simulink model "active_suspension_sim"  (R2020a)
settings: Solver=ode45  StartTime=0.0  StopTime=10.0  RelTol=1e-3
values from neighbouring files (symbols this model uses):
  A = [[-1/tau 0];[1/m -rho*CD*Af*x2e/m]]    [CruiseCtrl_StateFeedback_Int_design.m]    (also in CruiseCtrl_StateFeedback_Int_design_EJ6.m = Aaug; Driveline_ctrl_design.m = [-ds/(Jf*i^2) ds/(Jf*i) -cs/(Jf*i); Driveline_ctrl_design_accion_int.m = [-ds/(Jf*i^2) ds/(Jf*i) -cs/(Jf*i); active_suspension_ctrl_design.m = [[0 1 0 0 0];[-(cw+cs)/mw -ds/mw cs/mw ds/mw -1/mw];[0 0 0 1)
  B1 = [B H]    [CruiseCtrl_StateFeedback_Int_design.m]    (also in CruiseCtrl_StateFeedback_Int_design_EJ6.m = [Baug Haug]; Driveline_ctrl_design.m; Driveline_ctrl_design_accion_int.m; active_suspension_ctrl_design.m)
  C = [0 1]    [CruiseCtrl_StateFeedback_Int_design.m]    (also in CruiseCtrl_StateFeedback_Int_design_EJ6.m; Driveline_ctrl_design.m = eye(3); Driveline_ctrl_design_accion_int.m = eye(3); active_suspension_ctrl_design.m = [[-1 0 1 0 0];[cs/mc ds/mc -cs/mc -ds/mc 1/mc]])
  C1 = eye(2)    [CruiseCtrl_StateFeedback_Int_design.m]    (also in CruiseCtrl_StateFeedback_Int_design_EJ6.m = eye(3); active_suspension_ctrl_design.m = eye(5))
  D1 = zeros(2)    [CruiseCtrl_StateFeedback_Int_design.m]    (also in CruiseCtrl_StateFeedback_Int_design_EJ6.m = zeros(3); active_suspension_ctrl_design.m = zeros(5,2))
  K = acker(A,B,polos)    [CruiseCtrl_StateFeedback_Int_design.m]    (also in Driveline_ctrl_design.m; Driveline_ctrl_design_accion_int.m = Kaug(1, 1:3); active_suspension_ctrl_design.m = lqr(A,B,Qx,Qu))
settings Model: Creator=JonasMac  LastModifiedBy=Adriana
settings DataIOCC: LimitDataPoints=on  SaveFormat=Array  SignalLoggingSaveFormat=ModelDataLogs  ReturnWorkspaceOutputs=off
settings OptimizationCC: BlockReduction=off  BooleanDataType=off  LifeSpan=inf
settings DebuggingCC: SaveWithParameterizedLinksMsg=none  UnderspecifiedInitializationDetection=Classic  MergeDetectMultiDrivingBlocksExec=none  SignalResolutionControl=TryResolveAllWithWarning  MultiTaskDSMMsg=warning  MultiTaskCondExecSysMsg=none  SFUnexpectedBacktrackingDiag=warning  SFNoUnconditionalDefaultTransitionDiag=warning  SFExecutionAtInitializationDiag=none  ArithmeticOperatorsInVariantConditions=warning
settings HardwareCC: ProdBitPerPointer=32  ProdBitPerSizeT=32  ProdBitPerPtrDiffT=32  ProdLargestAtomicFloat=None  ProdIntDivRoundTo=Undefined  ProdEndianess=Unspecified  ProdWordSize=32  ProdHWDeviceType=32-bit Generic  TargetUnknown=on
settings ModelReferenceCC: PropagateSignalLabelsOutOfModel=off
settings SFSimCC: SimUseLocalCustomCode=off  CustomCodeUndefinedFunction=UseInterfaceOnly
settings RTWCC: RTWUseLocalCustomCode=off
settings CodeAppCC: StateflowObjectComments=on
settings GRTTargetCC: TargetLangStandard=C89/C90 (ANSI)
settings ConfigComp: CovMetricSettings=dw  CovHtmlReporting=on  CovSaveCumulativeToWorkspaceVar=on  CovSaveSingleToWorkspaceVar=on  CovExternalEMLEnable=off

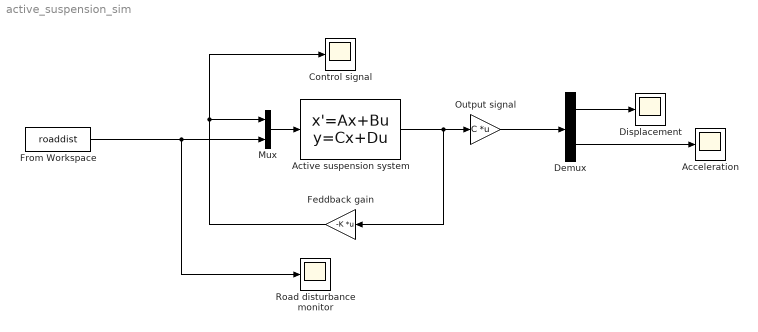
== system active_suspension_sim ==
  Acceleration : Scope
  Active suspension system : StateSpace  A=A  B=B1  C=C1  D=D1
  Control signal : Scope
  Demux : Demux  Outputs=2
  Displacement : Scope
  Feddback gain : Gain  Gain=-K  Multiplication=Matrix(K*u)
  From Workspace : FromWorkspace  VariableName=roaddist
  Mux : Mux  Inputs=2
  Output signal : Gain  Gain=C  Multiplication=Matrix(K*u)
  Road disturbance monitor : Scope
  wires:
  Demux/1 -> Displacement/1
  Active suspension system/1 -> Feddback gain/1, Output signal/1
  Feddback gain/1 -> Mux/1, Control signal/1
  Mux/1 -> Active suspension system/1
  Output signal/1 -> Demux/1
  Demux/2 -> Acceleration/1
  From Workspace/1 -> Road disturbance monitor/1, Mux/2
